simulink model "ddc_bpm_476_066"  (Simulink 7.8)
settings: Solver=ode45  StartTime=0.0  StopTime=2e-3  RelTol=1e-3
undefined symbols (not defined in the file): decim_factor_poly_35, dt_sim, frev_476, Fs_adc, n_ch, n_ovs, R_fofb, R_sec, R_sec_cfir, R_sec_pfir, xlipgetpartsetting
libraries: xbsIndex_r4 x1136, simulink x7
(part 3 of 10)

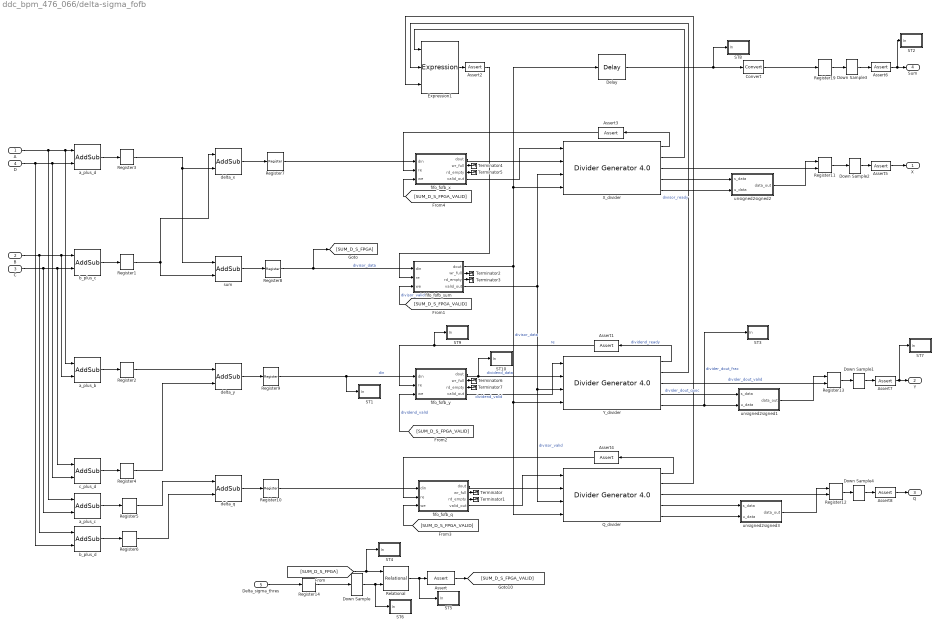
== system ddc_bpm_476_066/delta-sigma_fofb ==
  A : Inport
  B : Inport  Port=2
  C : Inport  Port=3
  D : Inport  Port=4
  Delta_sigma_thres : Inport  Port=5
  Assert{,5..8} (5 alike) : xbsIndex_r4/Assert  assert_type=off  type_source=Explicitly  gui_display_data_type=Fixed-point  arith_type="Signed  (2's comp)"  n_bits=16  bin_pt=14  preci_type=Single  exp_width=8  frac_width=24  assert_rate=on  rate_source=Explicitly  period=1/Fs_adc*R_fofb  output_port=on  block_type=assert
  Assert{1..4} (4 alike) : xbsIndex_r4/Assert  assert_type=off  type_source=Explicitly  gui_display_data_type=Fixed-point  arith_type="Signed  (2's comp)"  n_bits=16  bin_pt=14  preci_type=Single  exp_width=8  frac_width=24  assert_rate=on  rate_source=Explicitly  period=1/Fs_adc  output_port=on  block_type=assert
  Convert : xbsIndex_r4/Convert  gui_display_data_type=Fixed-point  arith_type="Signed  (2's comp)"  n_bits=25  bin_pt=21  float_type=Single  exp_bits=8  fraction_bits=24  quantization="Round  (unbiased: +/- Inf)"  overflow=Saturate  en=off  latency=0  dbl_ovrd=off  pipeline=off  block_type=convert
  Delay : xbsIndex_r4/Delay  rst=off  infoeditControl=Selection of Reset will increase slice count due to use of real FFs and instead of SRLs  en=off  latency=25  dbl_ovrd=off  reg_retiming=off  block_type=delay
  Down Sample{,1..4} (5 alike) : xbsIndex_r4/Down Sample  sample_ratio=R_fofb  sample_phase="Last Value of Frame  (most efficient)"  en=off  latency=1  dbl_ovrd=off  block_type=dsamp
  Expression1 : xbsIndex_r4/Expression  expression=a & b & c  align_bp=on  en=off  latency=0  precision=Full  arith_type=Unsigned  n_bits=16  bin_pt=0  dbl_ovrd=off  block_type=expr
  Q_divider : xbsIndex_r4/Divider Generator 4.0   algorithm_type=High_Radix  remainder_type=Fractional  fractional_width=24  clocks_per_division=1  divide_by_zero_detect=off  flowcontrol=NonBlocking  optimizegoal=Performance  latency_configuration=Manual  latency=25  dividend_has_tuser=off  dividend_has_tlast=off  divisor_has_tuser=off  divisor_has_tlast=off  aclken=off  aresetn=off  outtready=off  outtlastbehv=Null  trim_axipin_name=on  dividend_tuser_width=1  divisor_tuser_width=1  operand_sign=Signed  dividend_and_quotient_width=16  divisor_width=16  ip_name=Divider Generator  ip_version=4.0  dsptool_ready=true  ipcore_usecache=true  ipcore_useipmodelcache=true  wrapper_available=true  port_translation_map={'aclken' => 'en','aresetn' => 'rst'}  ipcore_fpga_part=xlipgetpartsetting(gcb, {'virtex7', 'xc7v1500t', '-2', 'fhg1157'})  ipcore_verbose=false  block_type=div_gen_v4_0
      settings: infoedit=Divider Generator 4.0
  Register{1..10,14,19} (12 alike) : xbsIndex_r4/Register  init=0  rst=off  en=off  dbl_ovrd=off  block_type=register
  Register11 : xbsIndex_r4/Register  init=0  rst=off  en=on  dbl_ovrd=off  block_type=register
  Register12 : xbsIndex_r4/Register  init=0  rst=off  en=on  dbl_ovrd=off  block_type=register
  Register13 : xbsIndex_r4/Register  init=0  rst=off  en=on  dbl_ovrd=off  block_type=register
  Relational : xbsIndex_r4/Relational  mode=a>b  en=off  latency=1  dbl_ovrd=off  block_type=relational
  ST1 : Subsystem
  ST10 : Subsystem
  ST2 : Subsystem
  ST3 : Subsystem
  ST4 : Subsystem
  ST5 : Subsystem
  ST6 : Subsystem
  ST7 : Subsystem
  ST8 : Subsystem
  ST9 : Subsystem
  Terminator{,1..7} (8 alike) : Terminator
  X_divider : xbsIndex_r4/Divider Generator 4.0   algorithm_type=High_Radix  remainder_type=Fractional  fractional_width=24  clocks_per_division=1  divide_by_zero_detect=off  flowcontrol=NonBlocking  optimizegoal=Performance  latency_configuration=Manual  latency=25  dividend_has_tuser=off  dividend_has_tlast=off  divisor_has_tuser=off  divisor_has_tlast=off  aclken=off  aresetn=off  outtready=off  outtlastbehv=Null  trim_axipin_name=on  dividend_tuser_width=1  divisor_tuser_width=1  operand_sign=Signed  dividend_and_quotient_width=16  divisor_width=16  ip_name=Divider Generator  ip_version=4.0  dsptool_ready=true  ipcore_usecache=true  ipcore_useipmodelcache=true  wrapper_available=true  port_translation_map={'aclken' => 'en','aresetn' => 'rst'}  ipcore_fpga_part=xlipgetpartsetting(gcb, {'virtex7', 'xc7v1500t', '-2', 'fhg1157'})  ipcore_verbose=false  block_type=div_gen_v4_0
      settings: infoedit=Divider Generator 4.0
  Y_divider : xbsIndex_r4/Divider Generator 4.0   algorithm_type=High_Radix  remainder_type=Fractional  fractional_width=24  clocks_per_division=1  divide_by_zero_detect=off  flowcontrol=NonBlocking  optimizegoal=Performance  latency_configuration=Manual  latency=25  dividend_has_tuser=off  dividend_has_tlast=off  divisor_has_tuser=off  divisor_has_tlast=off  aclken=off  aresetn=off  outtready=off  outtlastbehv=Null  trim_axipin_name=on  dividend_tuser_width=1  divisor_tuser_width=1  operand_sign=Signed  dividend_and_quotient_width=16  divisor_width=16  ip_name=Divider Generator  ip_version=4.0  dsptool_ready=true  ipcore_usecache=true  ipcore_useipmodelcache=true  wrapper_available=true  port_translation_map={'aclken' => 'en','aresetn' => 'rst'}  ipcore_fpga_part=xlipgetpartsetting(gcb, {'virtex7', 'xc7v1500t', '-2', 'fhg1157'})  ipcore_verbose=false  block_type=div_gen_v4_0
      settings: infoedit=Divider Generator 4.0
  a_plus_b : xbsIndex_r4/AddSub  mode=Addition  use_carryin=off  use_carryout=off  en=off  latency=0  precision=Full  arith_type=Unsigned  n_bits=16  bin_pt=14  quantization=Truncate  overflow=Wrap  dbl_ovrd=off  use_behavioral_HDL=off  hw_selection=Fabric  pipelined=off  block_type=addsub
  a_plus_c : xbsIndex_r4/AddSub  mode=Addition  use_carryin=off  use_carryout=off  en=off  latency=0  precision=Full  arith_type=Unsigned  n_bits=16  bin_pt=14  quantization=Truncate  overflow=Wrap  dbl_ovrd=off  use_behavioral_HDL=off  hw_selection=Fabric  pipelined=off  block_type=addsub
  a_plus_d : xbsIndex_r4/AddSub  mode=Addition  use_carryin=off  use_carryout=off  en=off  latency=0  precision=Full  arith_type=Unsigned  n_bits=16  bin_pt=14  quantization=Truncate  overflow=Wrap  dbl_ovrd=off  use_behavioral_HDL=off  hw_selection=Fabric  pipelined=off  block_type=addsub
  b_plus_c : xbsIndex_r4/AddSub  mode=Addition  use_carryin=off  use_carryout=off  en=off  latency=0  precision=Full  arith_type=Unsigned  n_bits=16  bin_pt=14  quantization=Truncate  overflow=Wrap  dbl_ovrd=off  use_behavioral_HDL=off  hw_selection=Fabric  pipelined=off  block_type=addsub
  b_plus_d : xbsIndex_r4/AddSub  mode=Addition  use_carryin=off  use_carryout=off  en=off  latency=0  precision=Full  arith_type=Unsigned  n_bits=16  bin_pt=14  quantization=Truncate  overflow=Wrap  dbl_ovrd=off  use_behavioral_HDL=off  hw_selection=Fabric  pipelined=off  block_type=addsub
  c_plus_d : xbsIndex_r4/AddSub  mode=Addition  use_carryin=off  use_carryout=off  en=off  latency=0  precision=Full  arith_type=Unsigned  n_bits=16  bin_pt=14  quantization=Truncate  overflow=Wrap  dbl_ovrd=off  use_behavioral_HDL=off  hw_selection=Fabric  pipelined=off  block_type=addsub
  delta_q : xbsIndex_r4/AddSub  mode=Subtraction  use_carryin=off  use_carryout=off  en=off  latency=0  precision=Full  arith_type=Unsigned  n_bits=16  bin_pt=14  quantization=Truncate  overflow=Wrap  dbl_ovrd=off  use_behavioral_HDL=off  hw_selection=Fabric  pipelined=off  block_type=addsub
  delta_x : xbsIndex_r4/AddSub  mode=Subtraction  use_carryin=off  use_carryout=off  en=off  latency=0  precision=Full  arith_type=Unsigned  n_bits=16  bin_pt=14  quantization=Truncate  overflow=Wrap  dbl_ovrd=off  use_behavioral_HDL=off  hw_selection=Fabric  pipelined=off  block_type=addsub
  delta_y : xbsIndex_r4/AddSub  mode=Subtraction  use_carryin=off  use_carryout=off  en=off  latency=0  precision=Full  arith_type=Unsigned  n_bits=16  bin_pt=14  quantization=Truncate  overflow=Wrap  dbl_ovrd=off  use_behavioral_HDL=off  hw_selection=Fabric  pipelined=off  block_type=addsub
  fifo_fofb_q : Subsystem
  fifo_fofb_sum : Subsystem
  fifo_fofb_x : Subsystem
  fifo_fofb_y : Subsystem
  sum : xbsIndex_r4/AddSub  mode=Addition  use_carryin=off  use_carryout=off  en=off  latency=0  precision=Full  arith_type=Unsigned  n_bits=16  bin_pt=14  quantization=Truncate  overflow=Wrap  dbl_ovrd=off  use_behavioral_HDL=off  hw_selection=Fabric  pipelined=off  block_type=addsub
  unsigned2signed1 : Subsystem
  unsigned2signed2 : Subsystem
  unsigned2signed3 : Subsystem
  X : Outport
  Y : Outport  Port=2
  Q : Outport  Port=3
  Sum : Outport  Port=4
  wires:
  A/1 -> a_plus_d/1, a_plus_b/1, a_plus_c/1
  D/1 -> a_plus_d/2, c_plus_d/2, b_plus_d/2
  B/1 -> b_plus_c/1, a_plus_b/2, b_plus_d/1
  C/1 -> b_plus_c/2, c_plus_d/1, a_plus_c/2
  a_plus_d/1 -> Register3/1
  b_plus_c/1 -> Register1/1
  a_plus_b/1 -> Register2/1
  c_plus_d/1 -> Register4/1
  a_plus_c/1 -> Register5/1
  b_plus_d/1 -> Register6/1
  Register3/1 -> sum/1, delta_x/2
  Register1/1 -> sum/2, delta_x/1
  Register2/1 -> delta_y/1
  Register4/1 -> delta_y/2
  Register5/1 -> delta_q/1
  Register6/1 -> delta_q/2
  delta_q/1 -> Register10/1
  delta_x/1 -> Register7/1
  Register19/1 -> Down Sample3/1
  Register8/1 -> [SUM_D_S_FPGA], fifo_fofb_sum/1(din)  "divisor_data"
  Register13/1 -> Down Sample1/1
  Register11/1 -> Down Sample2/1
  Register12/1 -> Down Sample4/1
  sum/1 -> Register8/1
  delta_y/1 -> Register9/1
  Delay/1 -> Convert/1, ST8/1(In)
  X_divider/3 -> Register11/2
  Register7/1 -> fifo_fofb_x/1(din)
  Y_divider/5 -> ST3/1(In), unsigned2signed1/2(u_data)  "divider_dout_frac"
  Y_divider/3 -> Register13/2  "divider_dout_valid"
  Q_divider/3 -> Register12/2
  Register9/1 -> ST1/1(In), fifo_fofb_y/1(din)  "din"
  Register10/1 -> fifo_fofb_q/1(din)
  X_divider/2 -> Expression1/1
  Y_divider/1 -> Assert1/1  "dividend_ready"
  Y_divider/2 -> Expression1/2  "divisor_ready"
  Delta_sigma_thres/1 -> Register14/1
  [SUM_D_S_FPGA] -> Relational/1, ST4/1(In)
  Relational/1 -> ST5/1(In), Assert/1
  fifo_fofb_x/1(dout) -> X_divider/2
  fifo_fofb_q/1(dout) -> Q_divider/2
  Q_divider/2 -> Expression1/3
  Q_divider/1 -> Assert4/1
  fifo_fofb_q/4(valid_out) -> Q_divider/1
  fifo_fofb_x/4(valid_out) -> X_divider/1
  X_divider/5 -> unsigned2signed2/2(u_data)
  X_divider/4 -> unsigned2signed2/1(s_data)
  unsigned2signed2/1(data_out) -> Register11/1
  Y_divider/4 -> unsigned2signed1/1(s_data)  "divider_dout_quoc"
  unsigned2signed1/1(data_out) -> Register13/1
  Q_divider/5 -> unsigned2signed3/2(u_data)
  Q_divider/4 -> unsigned2signed3/1(s_data)
  unsigned2signed3/1(data_out) -> Register12/1
  Convert/1 -> Register19/1
  fifo_fofb_sum/4(valid_out) -> Y_divider/3, Q_divider/3, X_divider/3  "divisor_valid"
  fifo_fofb_sum/1(dout) -> Y_divider/4, Q_divider/4, Delay/1, X_divider/4  "divisor_data"
  Assert/1 -> [SUM_D_S_FPGA_VALID]
  Down Sample/1 -> ST6/1(In), Relational/2
  fifo_fofb_y/1(dout) -> Y_divider/2, ST10/1(In)  "dividend_data"
  fifo_fofb_y/4(valid_out) -> Y_divider/1  "dividend_valid"
  Assert1/1 -> fifo_fofb_y/2(re), ST9/1(In)  "re"
  [SUM_D_S_FPGA_VALID] -> fifo_fofb_y/3(we)  "dividend_valid"
  [SUM_D_S_FPGA_VALID] -> fifo_fofb_sum/3(we)  "divisor_valid"
  Expression1/1 -> Assert2/1
  Assert2/1 -> fifo_fofb_sum/2(re)
  X_divider/1 -> Assert3/1
  Assert3/1 -> fifo_fofb_x/2(re)
  [SUM_D_S_FPGA_VALID] -> fifo_fofb_q/3(we)
  Assert4/1 -> fifo_fofb_q/2(re)
  [SUM_D_S_FPGA_VALID] -> fifo_fofb_x/3(we)
  Down Sample4/1 -> Assert8/1
  Down Sample1/1 -> Assert7/1
  Down Sample2/1 -> Assert5/1
  Down Sample3/1 -> Assert6/1
  Assert5/1 -> X/1
  Assert6/1 -> ST2/1(In), Sum/1
  Assert7/1 -> Y/1, ST7/1(In)
  Assert8/1 -> Q/1
  fifo_fofb_q/2(wr_full) -> Terminator/1
  fifo_fofb_q/3(rd_empty) -> Terminator1/1
  fifo_fofb_sum/2(wr_full) -> Terminator2/1
  fifo_fofb_sum/3(rd_empty) -> Terminator3/1
  fifo_fofb_x/2(wr_full) -> Terminator4/1
  fifo_fofb_x/3(rd_empty) -> Terminator5/1
  fifo_fofb_y/2(wr_full) -> Terminator6/1
  fifo_fofb_y/3(rd_empty) -> Terminator7/1
  Register14/1 -> Down Sample/1

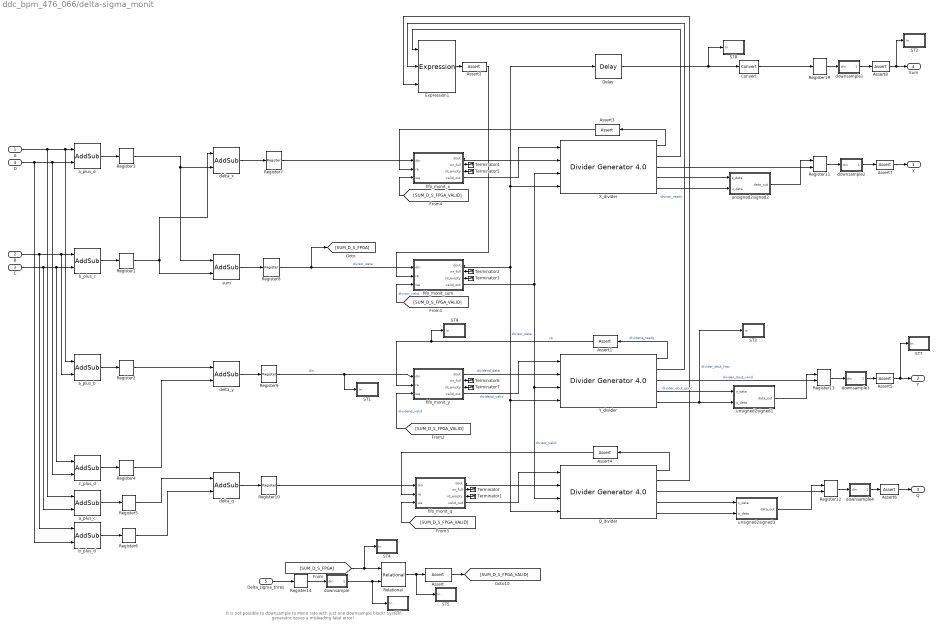
== system ddc_bpm_476_066/delta-sigma_monit ==
  note: It is not possible to downsample
      | to Monit rate with just one downsample block!
      | System generator issues a misleading fatal error!
  A : Inport
  B : Inport  Port=2
  C : Inport  Port=3
  D : Inport  Port=4
  Delta_sigma_thres : Inport  Port=5
  Assert{,5..8} (5 alike) : xbsIndex_r4/Assert  assert_type=off  type_source=Explicitly  gui_display_data_type=Fixed-point  arith_type="Signed  (2's comp)"  n_bits=16  bin_pt=14  preci_type=Single  exp_width=8  frac_width=24  assert_rate=on  rate_source=Explicitly  period=1/Fs_adc*(R_fofb*R_sec*R_sec_cfir*R_sec_pfir)  output_port=on  block_type=assert
  Assert{1..4} (4 alike) : xbsIndex_r4/Assert  assert_type=off  type_source=Explicitly  gui_display_data_type=Fixed-point  arith_type="Signed  (2's comp)"  n_bits=16  bin_pt=14  preci_type=Single  exp_width=8  frac_width=24  assert_rate=on  rate_source=Explicitly  period=1/Fs_adc*R_sec  output_port=on  block_type=assert
  Convert : xbsIndex_r4/Convert  gui_display_data_type=Fixed-point  arith_type="Signed  (2's comp)"  n_bits=25  bin_pt=21  float_type=Single  exp_bits=8  fraction_bits=24  quantization="Round  (unbiased: +/- Inf)"  overflow=Saturate  en=off  latency=0  dbl_ovrd=off  pipeline=off  block_type=convert
  Delay : xbsIndex_r4/Delay  rst=off  infoeditControl=Selection of Reset will increase slice count due to use of real FFs and instead of SRLs  en=off  latency=25  dbl_ovrd=off  reg_retiming=off  block_type=delay
  Expression1 : xbsIndex_r4/Expression  expression=a & b & c  align_bp=on  en=off  latency=0  precision=Full  arith_type=Unsigned  n_bits=16  bin_pt=0  dbl_ovrd=off  block_type=expr
  Q_divider : xbsIndex_r4/Divider Generator 4.0   algorithm_type=High_Radix  remainder_type=Fractional  fractional_width=24  clocks_per_division=1  divide_by_zero_detect=off  flowcontrol=NonBlocking  optimizegoal=Performance  latency_configuration=Manual  latency=25  dividend_has_tuser=off  dividend_has_tlast=off  divisor_has_tuser=off  divisor_has_tlast=off  aclken=off  aresetn=off  outtready=off  outtlastbehv=Null  trim_axipin_name=on  dividend_tuser_width=1  divisor_tuser_width=1  operand_sign=Signed  dividend_and_quotient_width=16  divisor_width=16  ip_name=Divider Generator  ip_version=4.0  dsptool_ready=true  ipcore_usecache=true  ipcore_useipmodelcache=true  wrapper_available=true  port_translation_map={'aclken' => 'en','aresetn' => 'rst'}  ipcore_fpga_part=xlipgetpartsetting(gcb, {'virtex7', 'xc7v1500t', '-2', 'fhg1157'})  ipcore_verbose=false  block_type=div_gen_v4_0
      settings: infoedit=Divider Generator 4.0
  Register{1..10,14,19} (12 alike) : xbsIndex_r4/Register  init=0  rst=off  en=off  dbl_ovrd=off  block_type=register
  Register11 : xbsIndex_r4/Register  init=0  rst=off  en=on  dbl_ovrd=off  block_type=register
  Register12 : xbsIndex_r4/Register  init=0  rst=off  en=on  dbl_ovrd=off  block_type=register
  Register13 : xbsIndex_r4/Register  init=0  rst=off  en=on  dbl_ovrd=off  block_type=register
  Relational : xbsIndex_r4/Relational  mode=a>b  en=off  latency=1  dbl_ovrd=off  block_type=relational
  ST1 : Subsystem
  ST2 : Subsystem
  ST3 : Subsystem
  ST4 : Subsystem
  ST5 : Subsystem
  ST6 : Subsystem
  ST7 : Subsystem
  ST8 : Subsystem
  ST9 : Subsystem
  Terminator{,1..7} (8 alike) : Terminator
  X_divider : xbsIndex_r4/Divider Generator 4.0   algorithm_type=High_Radix  remainder_type=Fractional  fractional_width=24  clocks_per_division=1  divide_by_zero_detect=off  flowcontrol=NonBlocking  optimizegoal=Performance  latency_configuration=Manual  latency=25  dividend_has_tuser=off  dividend_has_tlast=off  divisor_has_tuser=off  divisor_has_tlast=off  aclken=off  aresetn=off  outtready=off  outtlastbehv=Null  trim_axipin_name=on  dividend_tuser_width=1  divisor_tuser_width=1  operand_sign=Signed  dividend_and_quotient_width=16  divisor_width=16  ip_name=Divider Generator  ip_version=4.0  dsptool_ready=true  ipcore_usecache=true  ipcore_useipmodelcache=true  wrapper_available=true  port_translation_map={'aclken' => 'en','aresetn' => 'rst'}  ipcore_fpga_part=xlipgetpartsetting(gcb, {'virtex7', 'xc7v1500t', '-2', 'fhg1157'})  ipcore_verbose=false  block_type=div_gen_v4_0
      settings: infoedit=Divider Generator 4.0
  Y_divider : xbsIndex_r4/Divider Generator 4.0   algorithm_type=High_Radix  remainder_type=Fractional  fractional_width=24  clocks_per_division=1  divide_by_zero_detect=off  flowcontrol=NonBlocking  optimizegoal=Performance  latency_configuration=Manual  latency=25  dividend_has_tuser=off  dividend_has_tlast=off  divisor_has_tuser=off  divisor_has_tlast=off  aclken=off  aresetn=off  outtready=off  outtlastbehv=Null  trim_axipin_name=on  dividend_tuser_width=1  divisor_tuser_width=1  operand_sign=Signed  dividend_and_quotient_width=16  divisor_width=16  ip_name=Divider Generator  ip_version=4.0  dsptool_ready=true  ipcore_usecache=true  ipcore_useipmodelcache=true  wrapper_available=true  port_translation_map={'aclken' => 'en','aresetn' => 'rst'}  ipcore_fpga_part=xlipgetpartsetting(gcb, {'virtex7', 'xc7v1500t', '-2', 'fhg1157'})  ipcore_verbose=false  block_type=div_gen_v4_0
      settings: infoedit=Divider Generator 4.0
  a_plus_b : xbsIndex_r4/AddSub  mode=Addition  use_carryin=off  use_carryout=off  en=off  latency=0  precision=Full  arith_type=Unsigned  n_bits=16  bin_pt=14  quantization=Truncate  overflow=Wrap  dbl_ovrd=off  use_behavioral_HDL=off  hw_selection=Fabric  pipelined=off  block_type=addsub
  a_plus_c : xbsIndex_r4/AddSub  mode=Addition  use_carryin=off  use_carryout=off  en=off  latency=0  precision=Full  arith_type=Unsigned  n_bits=16  bin_pt=14  quantization=Truncate  overflow=Wrap  dbl_ovrd=off  use_behavioral_HDL=off  hw_selection=Fabric  pipelined=off  block_type=addsub
  a_plus_d : xbsIndex_r4/AddSub  mode=Addition  use_carryin=off  use_carryout=off  en=off  latency=0  precision=Full  arith_type=Unsigned  n_bits=16  bin_pt=14  quantization=Truncate  overflow=Wrap  dbl_ovrd=off  use_behavioral_HDL=off  hw_selection=Fabric  pipelined=off  block_type=addsub
  b_plus_c : xbsIndex_r4/AddSub  mode=Addition  use_carryin=off  use_carryout=off  en=off  latency=0  precision=Full  arith_type=Unsigned  n_bits=16  bin_pt=14  quantization=Truncate  overflow=Wrap  dbl_ovrd=off  use_behavioral_HDL=off  hw_selection=Fabric  pipelined=off  block_type=addsub
  b_plus_d : xbsIndex_r4/AddSub  mode=Addition  use_carryin=off  use_carryout=off  en=off  latency=0  precision=Full  arith_type=Unsigned  n_bits=16  bin_pt=14  quantization=Truncate  overflow=Wrap  dbl_ovrd=off  use_behavioral_HDL=off  hw_selection=Fabric  pipelined=off  block_type=addsub
  c_plus_d : xbsIndex_r4/AddSub  mode=Addition  use_carryin=off  use_carryout=off  en=off  latency=0  precision=Full  arith_type=Unsigned  n_bits=16  bin_pt=14  quantization=Truncate  overflow=Wrap  dbl_ovrd=off  use_behavioral_HDL=off  hw_selection=Fabric  pipelined=off  block_type=addsub
  delta_q : xbsIndex_r4/AddSub  mode=Subtraction  use_carryin=off  use_carryout=off  en=off  latency=0  precision=Full  arith_type=Unsigned  n_bits=16  bin_pt=14  quantization=Truncate  overflow=Wrap  dbl_ovrd=off  use_behavioral_HDL=off  hw_selection=Fabric  pipelined=off  block_type=addsub
  delta_x : xbsIndex_r4/AddSub  mode=Subtraction  use_carryin=off  use_carryout=off  en=off  latency=0  precision=Full  arith_type=Unsigned  n_bits=16  bin_pt=14  quantization=Truncate  overflow=Wrap  dbl_ovrd=off  use_behavioral_HDL=off  hw_selection=Fabric  pipelined=off  block_type=addsub
  delta_y : xbsIndex_r4/AddSub  mode=Subtraction  use_carryin=off  use_carryout=off  en=off  latency=0  precision=Full  arith_type=Unsigned  n_bits=16  bin_pt=14  quantization=Truncate  overflow=Wrap  dbl_ovrd=off  use_behavioral_HDL=off  hw_selection=Fabric  pipelined=off  block_type=addsub
  downsample : Subsystem
  downsample1 : Subsystem
  downsample2 : Subsystem
  downsample3 : Subsystem
  downsample4 : Subsystem
  fifo_monit_q : Subsystem
  fifo_monit_sum : Subsystem
  fifo_monit_x : Subsystem
  fifo_monit_y : Subsystem
  sum : xbsIndex_r4/AddSub  mode=Addition  use_carryin=off  use_carryout=off  en=off  latency=0  precision=Full  arith_type=Unsigned  n_bits=16  bin_pt=14  quantization=Truncate  overflow=Wrap  dbl_ovrd=off  use_behavioral_HDL=off  hw_selection=Fabric  pipelined=off  block_type=addsub
  unsigned2signed1 : Subsystem
  unsigned2signed2 : Subsystem
  unsigned2signed3 : Subsystem
  X : Outport
  Y : Outport  Port=2
  Q : Outport  Port=3
  Sum : Outport  Port=4
  wires:
  A/1 -> a_plus_d/1, a_plus_b/1, a_plus_c/1
  D/1 -> a_plus_d/2, c_plus_d/2, b_plus_d/2
  B/1 -> b_plus_c/1, a_plus_b/2, b_plus_d/1
  C/1 -> b_plus_c/2, c_plus_d/1, a_plus_c/2
  a_plus_d/1 -> Register3/1
  b_plus_c/1 -> Register1/1
  a_plus_b/1 -> Register2/1
  c_plus_d/1 -> Register4/1
  a_plus_c/1 -> Register5/1
  b_plus_d/1 -> Register6/1
  Register3/1 -> sum/1, delta_x/2
  Register1/1 -> sum/2, delta_x/1
  Register2/1 -> delta_y/1
  Register4/1 -> delta_y/2
  Register5/1 -> delta_q/1
  Register6/1 -> delta_q/2
  delta_q/1 -> Register10/1
  delta_x/1 -> Register7/1
  Register19/1 -> downsample1/1(din)
  Register8/1 -> [SUM_D_S_FPGA], fifo_monit_sum/1(din)  "divisor_data"
  Register13/1 -> downsample3/1(din)
  Register11/1 -> downsample2/1(din)
  Register12/1 -> downsample4/1(din)
  sum/1 -> Register8/1
  delta_y/1 -> Register9/1
  Delay/1 -> Convert/1, ST8/1(In)
  X_divider/3 -> Register11/2
  Register7/1 -> fifo_monit_x/1(din)
  Y_divider/5 -> ST3/1(In), unsigned2signed1/2(u_data)  "divider_dout_frac"
  Y_divider/3 -> Register13/2  "divider_dout_valid"
  Q_divider/3 -> Register12/2
  Register9/1 -> ST1/1(In), fifo_monit_y/1(din)  "din"
  Register10/1 -> fifo_monit_q/1(din)
  X_divider/2 -> Expression1/1
  Y_divider/1 -> Assert1/1  "dividend_ready"
  Y_divider/2 -> Expression1/2  "divisor_ready"
  Delta_sigma_thres/1 -> Register14/1
  [SUM_D_S_FPGA] -> Relational/1, ST4/1(In)
  Relational/1 -> ST5/1(In), Assert/1
  fifo_monit_x/1(dout) -> X_divider/2
  fifo_monit_q/1(dout) -> Q_divider/2
  Q_divider/2 -> Expression1/3
  Q_divider/1 -> Assert4/1
  fifo_monit_q/4(valid_out) -> Q_divider/1
  fifo_monit_x/4(valid_out) -> X_divider/1
  X_divider/5 -> unsigned2signed2/2(u_data)
  X_divider/4 -> unsigned2signed2/1(s_data)
  unsigned2signed2/1(data_out) -> Register11/1
  Y_divider/4 -> unsigned2signed1/1(s_data)  "divider_dout_quoc"
  unsigned2signed1/1(data_out) -> Register13/1
  Q_divider/5 -> unsigned2signed3/2(u_data)
  Q_divider/4 -> unsigned2signed3/1(s_data)
  unsigned2signed3/1(data_out) -> Register12/1
  Convert/1 -> Register19/1
  fifo_monit_sum/4(valid_out) -> Y_divider/3, Q_divider/3, X_divider/3  "divisor_valid"
  fifo_monit_sum/1(dout) -> Y_divider/4, Q_divider/4, Delay/1, X_divider/4  "divisor_data"
  Assert/1 -> [SUM_D_S_FPGA_VALID]
  downsample/1(dout) -> ST6/1(In), Relational/2
  fifo_monit_y/1(dout) -> Y_divider/2  "dividend_data"
  fifo_monit_y/4(valid_out) -> Y_divider/1  "dividend_valid"
  Assert1/1 -> fifo_monit_y/2(re), ST9/1(In)  "re"
  [SUM_D_S_FPGA_VALID] -> fifo_monit_y/3(we)  "dividend_valid"
  [SUM_D_S_FPGA_VALID] -> fifo_monit_sum/3(we)  "divisor_valid"
  Expression1/1 -> Assert2/1
  Assert2/1 -> fifo_monit_sum/2(re)
  X_divider/1 -> Assert3/1
  Assert3/1 -> fifo_monit_x/2(re)
  [SUM_D_S_FPGA_VALID] -> fifo_monit_q/3(we)
  Assert4/1 -> fifo_monit_q/2(re)
  [SUM_D_S_FPGA_VALID] -> fifo_monit_x/3(we)
  downsample1/1(dout) -> Assert8/1
  downsample2/1(dout) -> Assert7/1
  downsample3/1(dout) -> Assert5/1
  downsample4/1(dout) -> Assert6/1
  Assert6/1 -> Q/1
  Assert5/1 -> Y/1, ST7/1(In)
  Assert7/1 -> X/1
  Assert8/1 -> ST2/1(In), Sum/1
  fifo_monit_q/2(wr_full) -> Terminator/1
  fifo_monit_q/3(rd_empty) -> Terminator1/1
  fifo_monit_sum/2(wr_full) -> Terminator2/1
  fifo_monit_sum/3(rd_empty) -> Terminator3/1
  fifo_monit_x/2(wr_full) -> Terminator4/1
  fifo_monit_x/3(rd_empty) -> Terminator5/1
  fifo_monit_y/2(wr_full) -> Terminator6/1
  fifo_monit_y/3(rd_empty) -> Terminator7/1
  Register14/1 -> downsample/1(din)

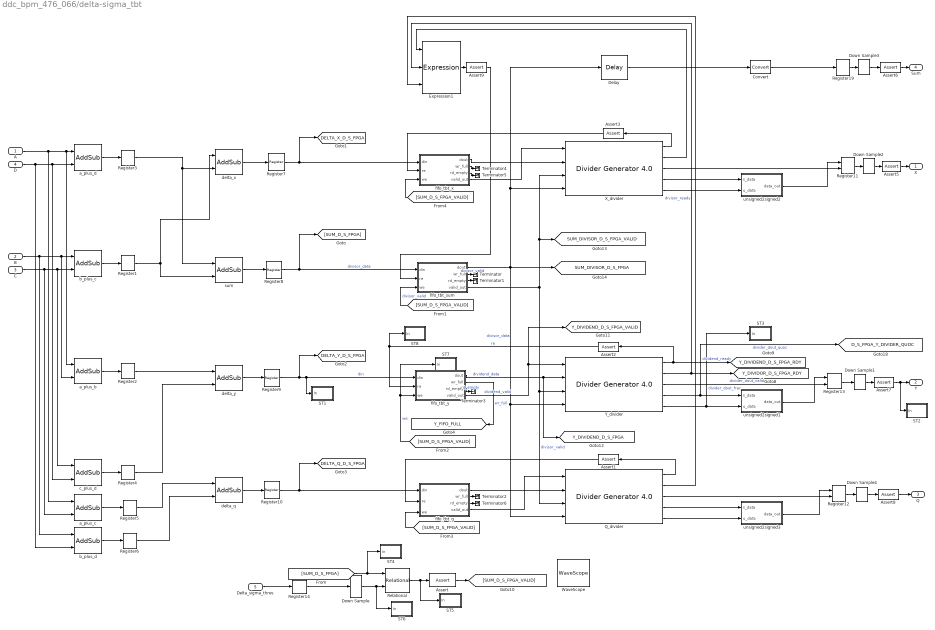
== system ddc_bpm_476_066/delta-sigma_tbt ==
  A : Inport
  B : Inport  Port=2
  C : Inport  Port=3
  D : Inport  Port=4
  Delta_sigma_thres : Inport  Port=5
  Assert{,5..8} (5 alike) : xbsIndex_r4/Assert  assert_type=off  type_source=Explicitly  gui_display_data_type=Fixed-point  arith_type="Signed  (2's comp)"  n_bits=16  bin_pt=14  preci_type=Single  exp_width=8  frac_width=24  assert_rate=on  rate_source=Explicitly  period=1/Fs_adc*decim_factor_poly_35  output_port=on  block_type=assert
  Assert{1..3,9} (4 alike) : xbsIndex_r4/Assert  assert_type=off  type_source=Explicitly  gui_display_data_type=Fixed-point  arith_type="Signed  (2's comp)"  n_bits=16  bin_pt=14  preci_type=Single  exp_width=8  frac_width=24  assert_rate=on  rate_source=Explicitly  period=1/Fs_adc  output_port=on  block_type=assert
  Convert : xbsIndex_r4/Convert  gui_display_data_type=Fixed-point  arith_type="Signed  (2's comp)"  n_bits=25  bin_pt=21  float_type=Single  exp_bits=8  fraction_bits=24  quantization="Round  (unbiased: +/- Inf)"  overflow=Saturate  en=off  latency=0  dbl_ovrd=off  pipeline=off  block_type=convert
  Delay : xbsIndex_r4/Delay  rst=off  infoeditControl=Selection of Reset will increase slice count due to use of real FFs and instead of SRLs  en=off  latency=25  dbl_ovrd=off  reg_retiming=off  block_type=delay
  Down Sample{,1..4} (5 alike) : xbsIndex_r4/Down Sample  sample_ratio=decim_factor_poly_35  sample_phase="Last Value of Frame  (most efficient)"  en=off  latency=1  dbl_ovrd=off  block_type=dsamp
  Expression1 : xbsIndex_r4/Expression  expression=a & b & c  align_bp=on  en=off  latency=0  precision=Full  arith_type=Unsigned  n_bits=16  bin_pt=0  dbl_ovrd=off  block_type=expr
  Q_divider : xbsIndex_r4/Divider Generator 4.0   algorithm_type=High_Radix  remainder_type=Fractional  fractional_width=24  clocks_per_division=1  divide_by_zero_detect=off  flowcontrol=NonBlocking  optimizegoal=Performance  latency_configuration=Manual  latency=25  dividend_has_tuser=off  dividend_has_tlast=off  divisor_has_tuser=off  divisor_has_tlast=off  aclken=off  aresetn=off  outtready=off  outtlastbehv=Null  trim_axipin_name=on  dividend_tuser_width=1  divisor_tuser_width=1  operand_sign=Signed  dividend_and_quotient_width=16  divisor_width=16  ip_name=Divider Generator  ip_version=4.0  dsptool_ready=true  ipcore_usecache=true  ipcore_useipmodelcache=true  wrapper_available=true  port_translation_map={'aclken' => 'en','aresetn' => 'rst'}  ipcore_fpga_part=xlipgetpartsetting(gcb, {'virtex7', 'xc7v1500t', '-2', 'fhg1157'})  ipcore_verbose=false  block_type=div_gen_v4_0
      settings: infoedit=Divider Generator 4.0
  Register{1..10,14,19} (12 alike) : xbsIndex_r4/Register  init=0  rst=off  en=off  dbl_ovrd=off  block_type=register
  Register11 : xbsIndex_r4/Register  init=0  rst=off  en=on  dbl_ovrd=off  block_type=register
  Register12 : xbsIndex_r4/Register  init=0  rst=off  en=on  dbl_ovrd=off  block_type=register
  Register13 : xbsIndex_r4/Register  init=0  rst=off  en=on  dbl_ovrd=off  block_type=register
  Relational : xbsIndex_r4/Relational  mode=a>b  en=off  latency=1  dbl_ovrd=off  block_type=relational
  ST1 : Subsystem
  ST2 : Subsystem
  ST3 : Subsystem
  ST4 : Subsystem
  ST5 : Subsystem
  ST6 : Subsystem
  ST7 : Subsystem
  ST8 : Subsystem
  Terminator{,1..6} (7 alike) : Terminator
  WaveScope : xbsIndex_r4/WaveScope  block_type=wavescope
  X_divider : xbsIndex_r4/Divider Generator 4.0   algorithm_type=High_Radix  remainder_type=Fractional  fractional_width=24  clocks_per_division=1  divide_by_zero_detect=off  flowcontrol=NonBlocking  optimizegoal=Performance  latency_configuration=Manual  latency=25  dividend_has_tuser=off  dividend_has_tlast=off  divisor_has_tuser=off  divisor_has_tlast=off  aclken=off  aresetn=off  outtready=off  outtlastbehv=Null  trim_axipin_name=on  dividend_tuser_width=1  divisor_tuser_width=1  operand_sign=Signed  dividend_and_quotient_width=16  divisor_width=16  ip_name=Divider Generator  ip_version=4.0  dsptool_ready=true  ipcore_usecache=true  ipcore_useipmodelcache=true  wrapper_available=true  port_translation_map={'aclken' => 'en','aresetn' => 'rst'}  ipcore_fpga_part=xlipgetpartsetting(gcb, {'virtex7', 'xc7v1500t', '-2', 'fhg1157'})  ipcore_verbose=false  block_type=div_gen_v4_0
      settings: infoedit=Divider Generator 4.0
  Y_divider : xbsIndex_r4/Divider Generator 4.0   algorithm_type=High_Radix  remainder_type=Fractional  fractional_width=24  clocks_per_division=1  divide_by_zero_detect=off  flowcontrol=NonBlocking  optimizegoal=Performance  latency_configuration=Manual  latency=25  dividend_has_tuser=off  dividend_has_tlast=off  divisor_has_tuser=off  divisor_has_tlast=off  aclken=off  aresetn=off  outtready=off  outtlastbehv=Null  trim_axipin_name=on  dividend_tuser_width=1  divisor_tuser_width=1  operand_sign=Signed  dividend_and_quotient_width=16  divisor_width=16  ip_name=Divider Generator  ip_version=4.0  dsptool_ready=true  ipcore_usecache=true  ipcore_useipmodelcache=true  wrapper_available=true  port_translation_map={'aclken' => 'en','aresetn' => 'rst'}  ipcore_fpga_part=xlipgetpartsetting(gcb, {'virtex7', 'xc7v1500t', '-2', 'fhg1157'})  ipcore_verbose=false  block_type=div_gen_v4_0
      settings: infoedit=Divider Generator 4.0
  a_plus_b : xbsIndex_r4/AddSub  mode=Addition  use_carryin=off  use_carryout=off  en=off  latency=0  precision=Full  arith_type=Unsigned  n_bits=16  bin_pt=14  quantization=Truncate  overflow=Wrap  dbl_ovrd=off  use_behavioral_HDL=off  hw_selection=Fabric  pipelined=off  block_type=addsub
  a_plus_c : xbsIndex_r4/AddSub  mode=Addition  use_carryin=off  use_carryout=off  en=off  latency=0  precision=Full  arith_type=Unsigned  n_bits=16  bin_pt=14  quantization=Truncate  overflow=Wrap  dbl_ovrd=off  use_behavioral_HDL=off  hw_selection=Fabric  pipelined=off  block_type=addsub
  a_plus_d : xbsIndex_r4/AddSub  mode=Addition  use_carryin=off  use_carryout=off  en=off  latency=0  precision=Full  arith_type=Unsigned  n_bits=16  bin_pt=14  quantization=Truncate  overflow=Wrap  dbl_ovrd=off  use_behavioral_HDL=off  hw_selection=Fabric  pipelined=off  block_type=addsub
  b_plus_c : xbsIndex_r4/AddSub  mode=Addition  use_carryin=off  use_carryout=off  en=off  latency=0  precision=Full  arith_type=Unsigned  n_bits=16  bin_pt=14  quantization=Truncate  overflow=Wrap  dbl_ovrd=off  use_behavioral_HDL=off  hw_selection=Fabric  pipelined=off  block_type=addsub
  b_plus_d : xbsIndex_r4/AddSub  mode=Addition  use_carryin=off  use_carryout=off  en=off  latency=0  precision=Full  arith_type=Unsigned  n_bits=16  bin_pt=14  quantization=Truncate  overflow=Wrap  dbl_ovrd=off  use_behavioral_HDL=off  hw_selection=Fabric  pipelined=off  block_type=addsub
  c_plus_d : xbsIndex_r4/AddSub  mode=Addition  use_carryin=off  use_carryout=off  en=off  latency=0  precision=Full  arith_type=Unsigned  n_bits=16  bin_pt=14  quantization=Truncate  overflow=Wrap  dbl_ovrd=off  use_behavioral_HDL=off  hw_selection=Fabric  pipelined=off  block_type=addsub
  delta_q : xbsIndex_r4/AddSub  mode=Subtraction  use_carryin=off  use_carryout=off  en=off  latency=0  precision=Full  arith_type=Unsigned  n_bits=16  bin_pt=14  quantization=Truncate  overflow=Wrap  dbl_ovrd=off  use_behavioral_HDL=off  hw_selection=Fabric  pipelined=off  block_type=addsub
  delta_x : xbsIndex_r4/AddSub  mode=Subtraction  use_carryin=off  use_carryout=off  en=off  latency=0  precision=Full  arith_type=Unsigned  n_bits=16  bin_pt=14  quantization=Truncate  overflow=Wrap  dbl_ovrd=off  use_behavioral_HDL=off  hw_selection=Fabric  pipelined=off  block_type=addsub
  delta_y : xbsIndex_r4/AddSub  mode=Subtraction  use_carryin=off  use_carryout=off  en=off  latency=0  precision=Full  arith_type=Unsigned  n_bits=16  bin_pt=14  quantization=Truncate  overflow=Wrap  dbl_ovrd=off  use_behavioral_HDL=off  hw_selection=Fabric  pipelined=off  block_type=addsub
  fifo_tbt_q : Subsystem
  fifo_tbt_sum : Subsystem
  fifo_tbt_x : Subsystem
  fifo_tbt_y : Subsystem
  sum : xbsIndex_r4/AddSub  mode=Addition  use_carryin=off  use_carryout=off  en=off  latency=0  precision=Full  arith_type=Unsigned  n_bits=16  bin_pt=14  quantization=Truncate  overflow=Wrap  dbl_ovrd=off  use_behavioral_HDL=off  hw_selection=Fabric  pipelined=off  block_type=addsub
  unsigned2signed1 : Subsystem
  unsigned2signed2 : Subsystem
  unsigned2signed3 : Subsystem
  X : Outport
  Y : Outport  Port=2
  Q : Outport  Port=3
  Sum : Outport  Port=4
  tag scope: DELTA_Q_D_S_FPGA=global, DELTA_X_D_S_FPGA=global, DELTA_Y_D_S_FPGA=global, D_S_FPGA_Y_DIVIDER_QUOC=global, SUM_DIVISOR_D_S_FPGA=global, SUM_DIVISOR_D_S_FPGA_VALID=global, Y_DIVIDEND_D_S_FPGA=global, Y_DIVIDEND_D_S_FPGA_RDY=global, Y_DIVIDEND_D_S_FPGA_VALID=global, Y_DIVIDOR_D_S_FPGA_RDY=global, Y_FIFO_FULL=global
  wires:
  A/1 -> a_plus_d/1, a_plus_b/1, a_plus_c/1
  D/1 -> a_plus_d/2, c_plus_d/2, b_plus_d/2
  B/1 -> b_plus_c/1, a_plus_b/2, b_plus_d/1
  C/1 -> b_plus_c/2, c_plus_d/1, a_plus_c/2
  a_plus_d/1 -> Register3/1
  b_plus_c/1 -> Register1/1
  a_plus_b/1 -> Register2/1
  c_plus_d/1 -> Register4/1
  a_plus_c/1 -> Register5/1
  b_plus_d/1 -> Register6/1
  Register3/1 -> sum/1, delta_x/2
  Register1/1 -> sum/2, delta_x/1
  Register2/1 -> delta_y/1
  Register4/1 -> delta_y/2
  Register5/1 -> delta_q/1
  Register6/1 -> delta_q/2
  delta_q/1 -> Register10/1
  delta_x/1 -> Register7/1
  Register19/1 -> Down Sample3/1
  Register8/1 -> [SUM_D_S_FPGA], fifo_tbt_sum/1(din)  "divisor_data"
  Register13/1 -> Down Sample1/1
  Register11/1 -> Down Sample2/1
  Register12/1 -> Down Sample4/1
  sum/1 -> Register8/1
  delta_y/1 -> Register9/1
  Delay/1 -> Convert/1
  X_divider/3 -> Register11/2
  Register7/1 -> [DELTA_X_D_S_FPGA], fifo_tbt_x/1(din)
  Y_divider/5 -> ST3/1(In), unsigned2signed1/2(u_data)  "divider_dout_frac"
  Y_divider/3 -> Register13/2  "divider_dout_valid"
  Q_divider/3 -> Register12/2
  Register9/1 -> [DELTA_Y_D_S_FPGA], ST1/1(In), fifo_tbt_y/1(din)  "din"
  Register10/1 -> [DELTA_Q_D_S_FPGA], fifo_tbt_q/1(din)
  X_divider/2 -> Expression1/1
  Y_divider/1 -> [Y_DIVIDEND_D_S_FPGA_RDY], Assert2/1  "dividend_ready"
  Y_divider/2 -> [Y_DIVIDOR_D_S_FPGA_RDY], Expression1/2  "divisor_ready"
  Delta_sigma_thres/1 -> Register14/1
  [SUM_D_S_FPGA] -> Relational/1, ST4/1(In)
  Relational/1 -> ST5/1(In), Assert/1
  fifo_tbt_x/1(dout) -> X_divider/2
  fifo_tbt_q/1(dout) -> Q_divider/2
  Q_divider/2 -> Expression1/3
  Q_divider/1 -> Assert1/1
  fifo_tbt_q/4(valid_out) -> Q_divider/1
  fifo_tbt_x/4(valid_out) -> X_divider/1
  X_divider/5 -> unsigned2signed2/2(u_data)
  X_divider/4 -> unsigned2signed2/1(s_data)
  unsigned2signed2/1(data_out) -> Register11/1
  Y_divider/4 -> [D_S_FPGA_Y_DIVIDER_QUOC], unsigned2signed1/1(s_data)  "divider_dout_quoc"
  unsigned2signed1/1(data_out) -> Register13/1
  Q_divider/5 -> unsigned2signed3/2(u_data)
  Q_divider/4 -> unsigned2signed3/1(s_data)
  unsigned2signed3/1(data_out) -> Register12/1
  Convert/1 -> Register19/1
  Assert/1 -> [SUM_D_S_FPGA_VALID]
  Down Sample/1 -> ST6/1(In), Relational/2
  fifo_tbt_y/1(dout) -> Y_divider/2, [Y_DIVIDEND_D_S_FPGA]  "dividend_data"
  fifo_tbt_y/2(wr_full) -> [Y_FIFO_FULL]  "wr_full"
  [SUM_D_S_FPGA_VALID] -> ST7/1(In), fifo_tbt_y/3(we)  "we"
  [SUM_D_S_FPGA_VALID] -> fifo_tbt_sum/3(we)  "divisor_valid"
  Expression1/1 -> Assert9/1
  Assert9/1 -> fifo_tbt_sum/2(re)
  [SUM_D_S_FPGA_VALID] -> fifo_tbt_x/3(we)
  X_divider/1 -> Assert3/1
  Assert3/1 -> fifo_tbt_x/2(re)
  [SUM_D_S_FPGA_VALID] -> fifo_tbt_q/3(we)
  Assert1/1 -> fifo_tbt_q/2(re)
  Down Sample1/1 -> Assert7/1
  Down Sample2/1 -> Assert5/1
  Down Sample3/1 -> Assert6/1
  Down Sample4/1 -> Assert8/1
  Assert6/1 -> Sum/1
  Assert5/1 -> X/1
  Assert7/1 -> Y/1, ST2/1(In)
  Assert8/1 -> Q/1
  Assert2/1 -> ST8/1(In), fifo_tbt_y/2(re)  "re"
  fifo_tbt_y/4(valid_out) -> Y_divider/1, [Y_DIVIDEND_D_S_FPGA_VALID]  "dividend_valid"
  fifo_tbt_sum/4(valid_out) -> Y_divider/3, Q_divider/3, X_divider/3, [SUM_DIVISOR_D_S_FPGA_VALID]  "divisor_valid"
  fifo_tbt_sum/2(wr_full) -> Terminator/1  "divisor_valid"
  fifo_tbt_sum/3(rd_empty) -> Terminator1/1
  fifo_tbt_x/2(wr_full) -> Terminator4/1
  fifo_tbt_x/3(rd_empty) -> Terminator5/1
  fifo_tbt_sum/1(dout) -> [SUM_DIVISOR_D_S_FPGA], Y_divider/4, Q_divider/4, X_divider/4, Delay/1  "divisor_data"
  fifo_tbt_q/2(wr_full) -> Terminator2/1
  fifo_tbt_q/3(rd_empty) -> Terminator6/1
  fifo_tbt_y/3(rd_empty) -> Terminator3/1  "rd_empty"
  Register14/1 -> Down Sample/1

== system ddc_bpm_476_066/monit_pos_1 ==
  din : Inport
  ch_in : Inport  Port=2
  Cast3 : Subsystem
  Delay1 : xbsIndex_r4/Delay  rst=off  infoeditControl=Selection of Reset will increase slice count due to use of real FFs and instead of SRLs  en=off  latency=2  dbl_ovrd=off  reg_retiming=off  block_type=delay
  Delay3 : xbsIndex_r4/Delay  rst=off  infoeditControl=Selection of Reset will increase slice count due to use of real FFs and instead of SRLs  en=off  latency=2  dbl_ovrd=off  reg_retiming=off  block_type=delay
  Register : xbsIndex_r4/Register  init=0  rst=off  en=off  dbl_ovrd=off  block_type=register
      settings: xl_area=[0, 0, 0, 0, 0, 0, 0]  block_version=VER_STRING_GOES_HERE
  Reinterpret : xbsIndex_r4/Reinterpret  force_arith_type=on  arith_type="Signed  (2's comp)"  force_bin_pt=on  bin_pt=20  block_type=reinterpret
  TDDM_monit_pos_1_out : Subsystem
  Terminator : Terminator
  Terminator1 : Terminator
  monit_pos_1_c : xbsIndex_r4/FIR Compiler 6.3   coefficientvector=hpoly_sec_1.Numerator  coefficient_sets=1  coefficient_reload=off  filter_type=Decimation  rate_change_type=Integer  interpolation_rate=1  decimation_rate=R_sec_poly_1  zero_pack_factor=1  channel_sequence=Basic  number_channels=4  pattern_list='P4-0,P4-1,P4-2,P4-3,P4-4'  number_paths=1  ratespecification=Hardware_Oversampling_Rate  sampleperiod=556  hardwareoversamplingrate=R_fofb*R_sec*R_sec_cfir*R_sec_pfir*n_ovs/n_ch  coefficient_sign=Signed  quantization=Quantize_Only  coefficient_width=16  bestprecision=on  coefficient_fractional_bits=18  coefficient_structure=Inferred  output_rounding_mode=Convergent_Rounding_to_Even  output_width=26  filter_architecture=Systolic_Multiply_Accumulate  optimization_goal=Area  data_buffer_type=Automatic  coefficient_buffer_type=Automatic  input_buffer_type=Automatic  output_buffer_type=Automatic  preference_for_other_storage=Automatic  multi_column_support=Automatic  columnconfig='1'  inter_column_pipe_length=4  data_has_tlast=Not_Required  m_data_has_tready=off  s_data_has_fifo=off  s_data_has_tuser=Chan_ID_Field  m_data_has_tuser=Chan_ID_Field  s_config_sync_mode=On_Vector  s_config_method=Single  num_reload_slots=1  has_aclken=off  has_aresetn=off  infoeditControl=ARESETn must be asserted for a minmum of 2 cycles  trim_axipin_name=on  passband_min=0.0  passband_max=0.5  stopband_min=0.5  stopband_max=1.0  filter_selection=1  gui_behaviour=Sysgen_GUI  data_sign=Signed  data_width=16  data_fractional_bits=0  data_tuser_width=1  wrapper_available=true  ip_wrap_arbitrary_binary_point=true  simulation_type=external_xfix  simulation_model=firv6_3_CModel:firv6_3_cmodel  ip_name=FIR Compiler  ip_version=6.3  dsptool_ready=true  ipcore_usecache=true  ipcore_useipmodelcache=true  ipcore_xco_need_fpga_part=true  port_translation_map={ 'aclken' => 'en', 'aresetn' => 'rst' }  run_core_at_system_period=true  ipcore_fpga_part=xlipgetpartsetting(gcb, {'virtex6', 'xc6vlx75t', '-3', 'ff784'})  block_type=fir_compiler_v6_3
      settings: infoedit=Maximum Possible : Maximizes oversampling rate. Abstracted input handshake (no s_data_tvalid) and automatic rate propagation.<br>Hardware Oversampling Rate : Specifies oversampling rate relative to the input sample period. Abstracted input handshake (no s_data_tvalid) and automatic rate propagation.<br>Sample Period : Specifies absolute oversampling rate. No input handshake abstraction (exposes s_data_tvalid) and no rate propagation.
  monit_1_pos_x : Outport
  monit_1_pos_y : Outport  Port=2
  monit_1_pos_q : Outport  Port=3
  monit_1_sum : Outport  Port=4
  wires:
  ch_in/1 -> Delay3/1
  monit_pos_1_c/1 -> Terminator/1
  monit_pos_1_c/2 -> Cast3/2(en)
  din/1 -> Delay1/1
  monit_pos_1_c/4 -> Cast3/1(data_in)
  monit_pos_1_c/3 -> Register/1
  Register/1 -> TDDM_monit_pos_1_out/2(monit_amp_ch_in)
  Cast3/1(out) -> TDDM_monit_pos_1_out/1(monit_amp_din)
  TDDM_monit_pos_1_out/4(monit_amp_data3_out) -> Reinterpret/1
  Reinterpret/1 -> monit_1_sum/1
  TDDM_monit_pos_1_out/3(monit_amp_data2_out) -> monit_1_pos_q/1
  TDDM_monit_pos_1_out/2(monit_amp_data1_out) -> monit_1_pos_y/1
  TDDM_monit_pos_1_out/1(monit_amp_data0_out) -> monit_1_pos_x/1
  monit_pos_1_c/5 -> Terminator1/1
  Delay3/1 -> monit_pos_1_c/1
  Delay1/1 -> monit_pos_1_c/2

== system ddc_bpm_476_066/BPF/ST5 ==
  In : Inport
  Display : Display
  Sample Time : xbsIndex_r4/Sample Time  block_type=sampletime
      settings: infoedit="The Sample Time block reports the normalized sample period of its input.  A signal's normalized sample period is not equivalent to its Simulink absolute sample period.<br><br>Hardware notes: This block is implemented as a constant in hardware."
  out : xbsIndex_r4/Gateway Out  inherit_from_input=on  hdl_port=off  timing_constraint=Data Rate  locs_specified=off  LOCs={}  UseAsDAC=off  DACChannel='1'  block_type=gatewayout
      settings: infoedit="Gateway out block.  Converts Xilinx fixed-point or floating-point type inputs into ouputs of type Simulink integer, single, double, or fixed point.<br><br>Hardware notes:  In hardware these blocks become top level output ports or are discarded, depending on how they are configured."
  wires:
  out/1 -> Display/1
  Sample Time/1 -> out/1
  In/1 -> Sample Time/1

== system ddc_bpm_476_066/FOFB_amp/ST1 ==
  In : Inport
  Display : Display
  Sample Time : xbsIndex_r4/Sample Time  block_type=sampletime
      settings: infoedit="The Sample Time block reports the normalized sample period of its input.  A signal's normalized sample period is not equivalent to its Simulink absolute sample period.<br><br>Hardware notes: This block is implemented as a constant in hardware."
  out : xbsIndex_r4/Gateway Out  inherit_from_input=on  hdl_port=off  timing_constraint=Data Rate  locs_specified=off  LOCs={}  UseAsDAC=off  DACChannel='1'  block_type=gatewayout
      settings: infoedit="Gateway out block.  Converts Xilinx fixed-point or floating-point type inputs into ouputs of type Simulink integer, single, double, or fixed point.<br><br>Hardware notes:  In hardware these blocks become top level output ports or are discarded, depending on how they are configured."
  wires:
  out/1 -> Display/1
  Sample Time/1 -> out/1
  In/1 -> Sample Time/1

== system ddc_bpm_476_066/FOFB_amp/ST5 ==
  In : Inport
  Display : Display
  Sample Time : xbsIndex_r4/Sample Time  block_type=sampletime
      settings: infoedit="The Sample Time block reports the normalized sample period of its input.  A signal's normalized sample period is not equivalent to its Simulink absolute sample period.<br><br>Hardware notes: This block is implemented as a constant in hardware."
  out : xbsIndex_r4/Gateway Out  inherit_from_input=on  hdl_port=off  timing_constraint=Data Rate  locs_specified=off  LOCs={}  UseAsDAC=off  DACChannel='1'  block_type=gatewayout
      settings: infoedit="Gateway out block.  Converts Xilinx fixed-point or floating-point type inputs into ouputs of type Simulink integer, single, double, or fixed point.<br><br>Hardware notes:  In hardware these blocks become top level output ports or are discarded, depending on how they are configured."
  wires:
  out/1 -> Display/1
  Sample Time/1 -> out/1
  In/1 -> Sample Time/1

== system ddc_bpm_476_066/FOFB_amp/TDDM_fofb_amp_4ch ==
  amp_in0 : Inport
  ch_in0 : Inport  Port=2
  amp_in1 : Inport  Port=3
  ch_in1 : Inport  Port=4
  TDDM_fofb_amp0 : Subsystem
  TDDM_fofb_amp1 : Subsystem
  Terminator : Terminator
  Terminator1 : Terminator
  amp_out0 : Outport
  amp_out1 : Outport  Port=2
  amp_out2 : Outport  Port=3
  amp_out3 : Outport  Port=4
  wires:
  amp_in0/1 -> TDDM_fofb_amp0/1(din)
  ch_in0/1 -> TDDM_fofb_amp0/2(ch_in)
  amp_in1/1 -> TDDM_fofb_amp1/1(din)
  TDDM_fofb_amp0/1(dout_ch0) -> amp_out0/1
  TDDM_fofb_amp0/2(dout_ch1) -> amp_out1/1
  TDDM_fofb_amp1/1(dout_ch0) -> amp_out2/1
  TDDM_fofb_amp1/2(dout_ch1) -> amp_out3/1
  TDDM_fofb_amp1/3(ch_out) -> Terminator/1
  TDDM_fofb_amp0/3(ch_out) -> Terminator1/1
  ch_in1/1 -> TDDM_fofb_amp1/2(ch_in)

== system ddc_bpm_476_066/FOFB_amp/fofb_amp0 ==
  Q_in : Inport
  I_in : Inport  Port=2
  ch_in : Inport  Port=3
  FOFB_CORDIC : Subsystem
  FOFB_amp : Subsystem
  amp_out : Outport
  phase_out : Outport  Port=2
  valid_out : Outport  Port=3
  ch_out : Outport  Port=4
  wires:
  FOFB_CORDIC/1(amp_out) -> amp_out/1
  FOFB_CORDIC/2(phase_out) -> phase_out/1
  FOFB_CORDIC/3(valid_out) -> valid_out/1
  FOFB_CORDIC/4(ch_out) -> ch_out/1
  FOFB_amp/4(ch_out) -> FOFB_CORDIC/4(ch_in)
  FOFB_amp/3(valid_out) -> FOFB_CORDIC/3(valid_in)
  FOFB_amp/2(I_out) -> FOFB_CORDIC/2(I_in)
  FOFB_amp/1(Q_out) -> FOFB_CORDIC/1(Q_in)
  Q_in/1 -> FOFB_amp/1(Q_in)
  I_in/1 -> FOFB_amp/2(I_in)
  ch_in/1 -> FOFB_amp/3(ch_in)

== system ddc_bpm_476_066/FOFB_amp/fofb_amp1 ==
  Q_in : Inport
  I_in : Inport  Port=2
  ch_in : Inport  Port=3
  FOFB_CORDIC : Subsystem
  FOFB_amp : Subsystem
  amp_out : Outport
  phase_out : Outport  Port=2
  valid_out : Outport  Port=3
  ch_out : Outport  Port=4
  wires:
  FOFB_CORDIC/1(amp_out) -> amp_out/1
  FOFB_CORDIC/2(phase_out) -> phase_out/1
  FOFB_CORDIC/3(valid_out) -> valid_out/1
  FOFB_CORDIC/4(ch_out) -> ch_out/1
  FOFB_amp/4(ch_out) -> FOFB_CORDIC/4(ch_in)
  FOFB_amp/3(valid_out) -> FOFB_CORDIC/3(valid_in)
  FOFB_amp/2(I_out) -> FOFB_CORDIC/2(I_in)
  FOFB_amp/1(Q_out) -> FOFB_CORDIC/1(Q_in)
  Q_in/1 -> FOFB_amp/1(Q_in)
  I_in/1 -> FOFB_amp/2(I_in)
  ch_in/1 -> FOFB_amp/3(ch_in)

== system ddc_bpm_476_066/Ksum_fofb_mult/Cast_truncate1 ==
  In1 : Inport
  Reinterpret : xbsIndex_r4/Reinterpret  force_arith_type=on  arith_type="Signed  (2's comp)"  force_bin_pt=on  bin_pt=20  block_type=reinterpret
  Slice : xbsIndex_r4/Slice  nbits=26  boolean_output=off  mode=Upper Bit Location + Width  bit1=0  base1=MSB of Input  bit0=0  base0=LSB of Input  dbl_ovrd=off  block_type=slice
  Out1 : Outport
  wires:
  Slice/1 -> Reinterpret/1
  Reinterpret/1 -> Out1/1
  In1/1 -> Slice/1

== system ddc_bpm_476_066/Ksum_tbt_mult1/Cast_truncate1 ==
  In1 : Inport
  Reinterpret : xbsIndex_r4/Reinterpret  force_arith_type=on  arith_type="Signed  (2's comp)"  force_bin_pt=on  bin_pt=20  block_type=reinterpret
  Slice : xbsIndex_r4/Slice  nbits=26  boolean_output=off  mode=Upper Bit Location + Width  bit1=0  base1=MSB of Input  bit0=0  base0=LSB of Input  dbl_ovrd=off  block_type=slice
  Out1 : Outport
  wires:
  Slice/1 -> Reinterpret/1
  Reinterpret/1 -> Out1/1
  In1/1 -> Slice/1

== system ddc_bpm_476_066/Ksum_tbt_mult2/Cast_truncate1 ==
  In1 : Inport
  Reinterpret : xbsIndex_r4/Reinterpret  force_arith_type=on  arith_type="Signed  (2's comp)"  force_bin_pt=on  bin_pt=20  block_type=reinterpret
  Slice : xbsIndex_r4/Slice  nbits=26  boolean_output=off  mode=Upper Bit Location + Width  bit1=0  base1=MSB of Input  bit0=0  base0=LSB of Input  dbl_ovrd=off  block_type=slice
  Out1 : Outport
  wires:
  Slice/1 -> Reinterpret/1
  Reinterpret/1 -> Out1/1
  In1/1 -> Slice/1

== system ddc_bpm_476_066/Ksum_tbt_mult3/Cast_truncate1 ==
  In1 : Inport
  Reinterpret : xbsIndex_r4/Reinterpret  force_arith_type=on  arith_type="Signed  (2's comp)"  force_bin_pt=on  bin_pt=20  block_type=reinterpret
  Slice : xbsIndex_r4/Slice  nbits=26  boolean_output=off  mode=Upper Bit Location + Width  bit1=0  base1=MSB of Input  bit0=0  base0=LSB of Input  dbl_ovrd=off  block_type=slice
  Out1 : Outport
  wires:
  Slice/1 -> Reinterpret/1
  Reinterpret/1 -> Out1/1
  In1/1 -> Slice/1

== system ddc_bpm_476_066/Kx_fofb_mult/Cast_truncate1 ==
  In1 : Inport
  Reinterpret : xbsIndex_r4/Reinterpret  force_arith_type=on  arith_type="Signed  (2's comp)"  force_bin_pt=on  bin_pt=0  block_type=reinterpret
  Slice : xbsIndex_r4/Slice  nbits=26  boolean_output=off  mode=Upper Bit Location + Width  bit1=0  base1=MSB of Input  bit0=0  base0=LSB of Input  dbl_ovrd=off  block_type=slice
  Out1 : Outport
  wires:
  Slice/1 -> Reinterpret/1
  Reinterpret/1 -> Out1/1
  In1/1 -> Slice/1

== system ddc_bpm_476_066/Kx_monit_mult/Cast_truncate1 ==
  In1 : Inport
  Reinterpret : xbsIndex_r4/Reinterpret  force_arith_type=on  arith_type="Signed  (2's comp)"  force_bin_pt=on  bin_pt=0  block_type=reinterpret
  Slice : xbsIndex_r4/Slice  nbits=26  boolean_output=off  mode=Upper Bit Location + Width  bit1=0  base1=MSB of Input  bit0=0  base0=LSB of Input  dbl_ovrd=off  block_type=slice
  Out1 : Outport
  wires:
  Slice/1 -> Reinterpret/1
  Reinterpret/1 -> Out1/1
  In1/1 -> Slice/1

== system ddc_bpm_476_066/Kx_monit_mult1/Cast_truncate1 ==
  In1 : Inport
  Reinterpret : xbsIndex_r4/Reinterpret  force_arith_type=on  arith_type="Signed  (2's comp)"  force_bin_pt=on  bin_pt=0  block_type=reinterpret
  Slice : xbsIndex_r4/Slice  nbits=26  boolean_output=off  mode=Upper Bit Location + Width  bit1=0  base1=MSB of Input  bit0=0  base0=LSB of Input  dbl_ovrd=off  block_type=slice
  Out1 : Outport
  wires:
  Slice/1 -> Reinterpret/1
  Reinterpret/1 -> Out1/1
  In1/1 -> Slice/1
